simulink model "AngularFlight_TestModel"  (R2014a)
settings: Solver=ode45  StartTime=0.0  StopTime=10.0  RelTol=1e-3
undefined symbols (not defined in the file or in its folder): center_of_pressure, factstruct
libraries: aerolibadyn x2, rocket_dynamic_data_library x2, aerolibbdyn x2, aerolib6dof2 x1, rocket_angular_flight_library x1, aerolibasang x1
settings Model: Creator=scorpii  LastModifiedBy=scorpii

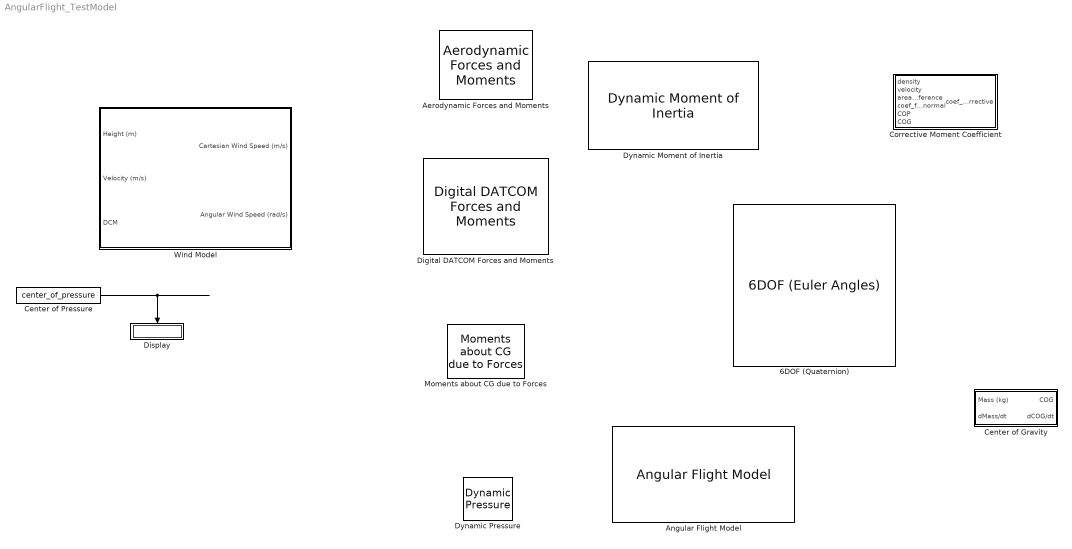
== system AngularFlight_TestModel ==
  6DOF (Quaternion) : aerolib6dof2/6DOF (Euler Angles)  units=Metric (MKS)  mtype=Fixed  rep=Quaternion  xme_0=[0 0 0]  Vm_0=[0 0 0]  eul_0=[0 0 0]  pm_0=[0 0 0]  mass_0=1.0  mass_e=0.5  mass_f=2.0  inertia=eye(3)  inertia_e=eye(3)  inertia_f=2*eye(3)  k_quat=1.0  vre_flag=on
  "Aerodynamic Forces and Moments " : aerolibadyn/Aerodynamic Forces and Moments   inputAxes=Body  outputForceAxes=Body  outputMomentAxes=Body  S=1  b=1  cbar=1
  Angular Flight Model : rocket_angular_flight_library/Angular Flight Model
  Center of Gravity : Subsystem
  Center of Pressure : Constant  Value=center_of_pressure
  Corrective Moment Coefficient : Subsystem
  Digital DATCOM Forces and Moments : aerolibadyn/Digital DATCOM Forces and Moments  units=Metric (MKS)  dcase=factstruct{1}  fmode=Body  buildno=0  imethod=Linear  emethod=Linear  rmethod=Linear Extrapolation  action=None
  Display : Display
  Dynamic Moment of Inertia : rocket_dynamic_data_library/Dynamic Moment of Inertia
  Dynamic Pressure : aerolibasang/Dynamic Pressure
  Moments about CG due to Forces : aerolibbdyn/Moments about CG  due to Forces
  Wind Model : Subsystem
  wires:
  Center of Pressure/1 -> Display/1

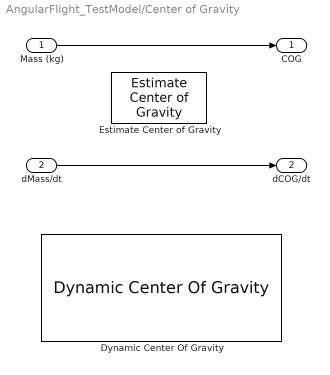
== system AngularFlight_TestModel/Center of Gravity ==
  Mass (kg) : Inport
  dMass/dt : Inport  Port=2
  Dynamic Center Of Gravity : rocket_dynamic_data_library/Dynamic Center Of Gravity
  Estimate Center of Gravity : aerolibbdyn/Estimate Center of Gravity  fmass=2  emass=1  fcg=[1 1 1]'  ecg=[0.5 0.5 0.5]'
  COG : Outport
  dCOG/dt : Outport  Port=2
  wires:
  Mass (kg)/1 -> COG/1
  dMass/dt/1 -> dCOG/dt/1

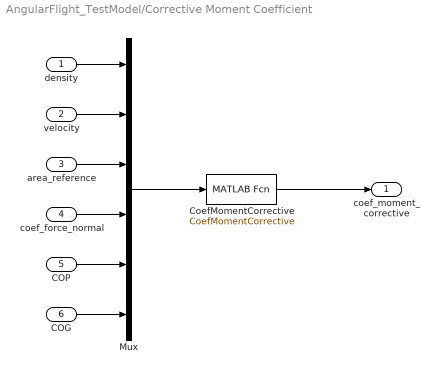
== system AngularFlight_TestModel/Corrective Moment Coefficient ==
  density : Inport
  velocity : Inport  Port=2
  area_reference : Inport  Port=3
  coef_force_normal : Inport  Port=4
  COP : Inport  Port=5
  COG : Inport  Port=6
  CoefMomentCorrective : MATLABFcn  MATLABFcn=CoefMomentCorrective
  Mux : Mux  Inputs=6
  coef_moment_corrective : Outport
  wires:
  density/1 -> Mux/1
  velocity/1 -> Mux/2
  area_reference/1 -> Mux/3
  coef_force_normal/1 -> Mux/4
  COP/1 -> Mux/5
  COG/1 -> Mux/6
  Mux/1 -> CoefMomentCorrective/1
  CoefMomentCorrective/1 -> coef_moment_corrective/1

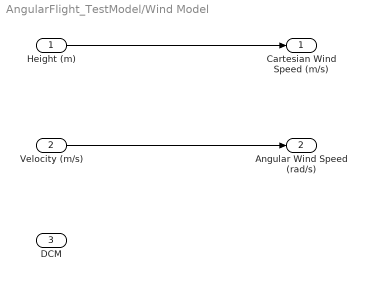
== system AngularFlight_TestModel/Wind Model ==
  Height (m) : Inport
  Velocity (m/s) : Inport  Port=2
  DCM : Inport  Port=3
  Cartesian Wind Speed (m/s) : Outport
  Angular Wind Speed (rad/s) : Outport  Port=2
  wires:
  Height (m)/1 -> Cartesian Wind Speed (m/s)/1
  Velocity (m/s)/1 -> Angular Wind Speed (rad/s)/1
